simulink model "clase_008_codigo_001"  (R2024a)
settings: Solver=VariableStepAuto  StartTime=0.0  StopTime=10.0  RelTol=1e-3
undefined symbols (not defined in the file): magnitude

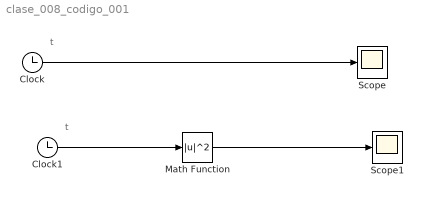
== system clase_008_codigo_001 ==
  note: t
  note: t
  Clock : Clock
  Clock1 : Clock
  Math Function : Math  Operator=magnitude^2
  Scope : Scope
  Scope1 : Scope
  wires:
  Clock/1 -> Scope/1
  Clock1/1 -> Math Function/1
  Math Function/1 -> Scope1/1
